simulink model "CurrentWithSim"  (R2022b)
settings: Solver=VariableStepAuto  StartTime=0.0  StopTime=20  RelTol=1e-3
PreLoadFcn:
  | openManipulatorParameters;
PostLoadFcn:
  | % Insert Communication Stuff Here
StartFcn:
  | myDxl.doEnableTorque(11);
  | myDxl.doEnableTorque(12);
  | myDxl.doEnableTorque(13);
  | myDxl.doEnableTorque(14);
  | myDxl.doEnableTorque(15);
StopFcn:
  | myDxl.doDisableTorque(11);
  | myDxl.doDisableTorque(12);
  | myDxl.doDisableTorque(13);
  | myDxl.doDisableTorque(14);
  | myDxl.doDisableTorque(15);
undefined symbols (not defined in the file): TsCtrl
libraries: slDxl_lib x12, OpenManipulatorLib x3, sm_lib x2, nesl_utility x1
CloseFcn:
  | myDxl.delete()
settings Model: Creator=scastro  LastModifiedBy=Boog
settings SolverCC: AlgebraicLoopSolver=TrustRegion  DecoupledContinuousIntegration=on  MinimalZcImpactIntegration=on
settings DataIOCC: ReturnWorkspaceOutputs=off
settings DebuggingCC: UnconnectedInputMsg=warning  UnconnectedOutputMsg=warning  UnconnectedLineMsg=warning  SFMachineParentedDataDiag=warning  ArithmeticOperatorsInVariantConditions=warning
settings ModelReferenceCC: EnableRefExpFcnMdlSchedulingChecks=on
settings SFSimCC: SimUseLocalCustomCode=off  CustomCodeUndefinedFunction=UseInterfaceOnly
settings RTWCC: RTWUseLocalCustomCode=off
settings ExplorerConfigSet: InternalSimMechanicsExplorerSettings="<ExplorerConfiguration><canonicalview>default</canonicalview><AnimationSetting><BasePlaybackSpeed>1.0</BasePlaybackSpeed><PlaybackSpeedFactor>1.0</PlaybackSpeedFactor></AnimationSetting><TilePanel><TileInfo><Tiles Columns=\"1\" Count=\"1\" Rows=\"1\"><Column Weight=\"1\"/><Row Weight=\"1\"/><Tile Height=\"1\" Width=\"1\" X=\"0\" Y=\"0\"/></Tiles></TileInfo><SceneInfo><SceneViewer><BGColor><R>0.60000002384185791</R><G>0.60000002384185791</G><B>0.60000002384185791</B></BGColor><Camera><DoPerspective>off</DoPerspective><Position><X>0.428752942017998073</X><Y>-0.712150369953937545</Y><Z>0.628314823463847372</Z></Position><Center><X>0.0455703138120887447</X><Y>0.0802507835591396851</Y><Z>0.153687090021758288</Z></Center><Up><X>-0.128866037345358619</X><Y>0.462960972240881619</Y><Z>0.876961049648547597</Z></Up><ViewLimDist>1</ViewLimDist><YLim>0.579070269035580121</YLim><XLim>0.64437894599448009</XLim></Camera></SceneViewer></SceneInfo></TilePanel><MechEditorPanel><Cameras/><GfxPanelCameraMap/><VideoCreator><PlaybackSpeedRatio>1.0</PlaybackSpeedRatio><FrameRate>30</FrameRate><VideoFormat>Motion JPEG AVI</VideoFormat><FrameSize>auto</FrameSize></VideoCreator></MechEditorPanel></ExplorerConfiguration>"

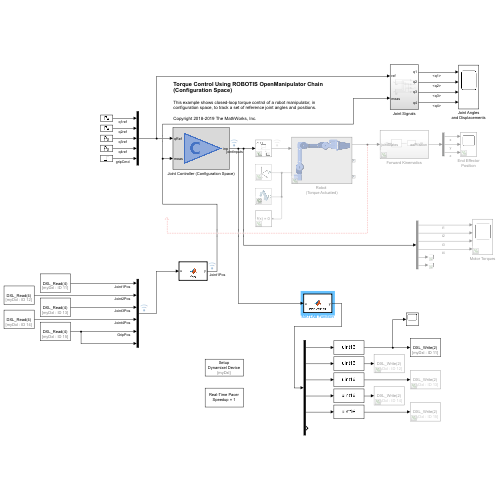
[thumbnail: Simulink's stored preview of the top-level diagram]
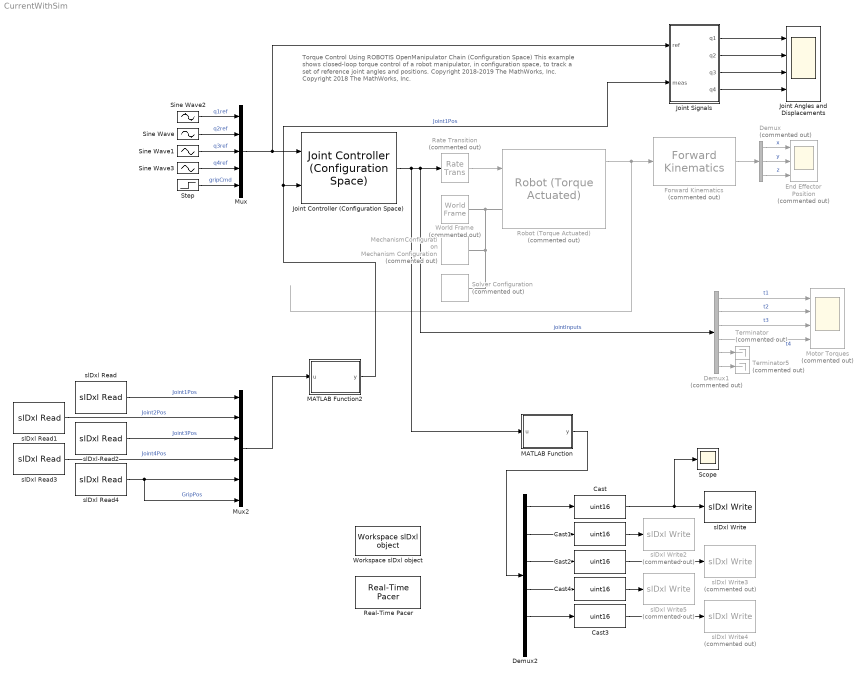
== system CurrentWithSim ==
  note: Torque Control Using ROBOTIS OpenManipulator Chain (Configuration Space)
      |
      | This example shows closed-loop torque control of a robot manipulator, in configuration space, to track a set of reference joint angles and positions.
      |
      | Copyright 2018-2019 The MathWorks, Inc.
      |
      | Copyright 2018 The MathWorks, Inc.
  Cast{,1..4} (5 alike) : DataTypeConversion  OutDataTypeStr=uint16  SaturateOnIntegerOverflow=off  RndMeth=Floor
  Demux : Demux  Commented=on  Outputs=3
  Demux1 : Demux  Commented=on  Outputs=6
  Demux2 : Demux  Outputs=6
  End Effector Position : Scope  Commented=on  NumInputPorts=3
  Forward Kinematics : OpenManipulatorLib/Forward Kinematics  Commented=on  SystemSampleTime=-1  VariantActivationTime=update diagram  Latency=0  AutoFrameSizeCalculation=off
  Joint Angles and Displacements : Scope  NumInputPorts=4
  Joint Controller (Configuration Space) : OpenManipulatorLib/Joint Controller (Configuration Space)  SystemSampleTime=-1  VariantControl=ctrlType==1  VariantActivationTime=update diagram  Latency=0  AutoFrameSizeCalculation=off
  Joint Signals : Subsystem
  MATLAB Function : MATLAB Function  TreatAsAtomicUnit=on
  MATLAB Function2 : MATLAB Function  TreatAsAtomicUnit=on
  MechanismConfiguration : sm_lib/Utilities/Mechanism Configuration  Commented=on  UniformGravity=Constant  GravityVector=[0 0 -9.80665]  GravityUnits=m/s^2  LinearizationDelta=0.001  JointModeTransitionNonlinearIterations=2
  Motor Torques : Scope  Commented=on  NumInputPorts=4
  Mux : Mux  Inputs=5
  Mux2 : Mux  Inputs=6
  Rate Transition : RateTransition  Commented=on
  Real-Time Pacer : slDxl_lib/Real-Time Pacer  simTimePerRealTime=1
  Robot (Torque Actuated) : OpenManipulatorLib/Robot  (Torque Actuated)  Commented=on  SystemSampleTime=-1  VariantActivationTime=update diagram  Latency=0  AutoFrameSizeCalculation=off
  Scope : Scope
  Sine Wave : Sin  Amplitude=pi/4  Frequency=0.6  SampleTime=TsCtrl
  Sine Wave1 : Sin  Amplitude=pi/4  Frequency=1.5  SampleTime=TsCtrl
  Sine Wave2 : Sin  Amplitude=2*pi/3  Frequency=0.4  SampleTime=TsCtrl
  Sine Wave3 : Sin  Amplitude=pi/3  SampleTime=TsCtrl
  Solver Configuration : nesl_utility/Solver Configuration  Commented=on  PhysicalDomain=network_engine_domain  SubClassName=solver  LeftPortType=input  RightPortType=generic  Tones=[]  Harmonics=[]  SimulateNoise=off  Profile=off  UseLocalSampling=off  EnableSwitchedLinearOptims=on  FrequencyDomain=off  UseCCode=off  RelTol=0.001  AbsTol=1e-06  MinStep=1e-09  ToWorkspace=off  RevertToSquareIcSolve=off  NumHomotopyIterations=100  PhasorMode=off  PhasorModeNumHarmonics=1  ConsistencySolver=NEWTON_FTOL  IndexReductionMethod=DerivativeReplacement  DoDC=off  ResidualTolerance=1e-09  ConsistencyTolSource=GLOBAL  ConsistencyAbsTol=0.001  ConsistencyRelTol=0.001  ConsistencyTolFactor=0.001  UseLocalSolver=off  LocalSolverChoice=NE_BACKWARD_EULER_ADVANCER  ResolveIndetEquations=on  FunctionEvalNumThread=1  LocalSolverSampleTime=0.001  DoFixedCost=off  MaxNonlinIter=3  MaxModeIter=2  ComputeImpulses=off  ImpulseIterations=2  LinearAlgebra=Sparse  LinearAlgebraNumThread=0  EquationFormulation=NE_TIME_EF  DelaysMemoryBudget=1024  AutomaticFiltering=on  FilteringTimeConstant=0.001  PartitionStorageMethod=AS_NEEDED  PartitionMemoryBudget=1024  PartitionMethod=FAST
  Step : Step  Time=5  SampleTime=TsCtrl
  Terminator : Terminator  Commented=on
  Terminator5 : Terminator  Commented=on
  Workspace slDxl object : slDxl_lib/Workspace slDxl object  slDxlVarName=Existing Object Handle #1  workspaceVarName=myDxl
  World Frame : sm_lib/Frames and Transforms/World Frame  Commented=on
  slDxl Read : slDxl_lib/slDxl Read  slDxlObject=Existing Object Handle #1  DXL_ID=11  DXL_ADDR=132  DXL_READ_SIZE=4  sampleT=Ts
  slDxl Read1 : slDxl_lib/slDxl Read  slDxlObject=Existing Object Handle #1  DXL_ID=12  DXL_ADDR=132  DXL_READ_SIZE=4  sampleT=Ts
  slDxl Read2 : slDxl_lib/slDxl Read  slDxlObject=Existing Object Handle #1  DXL_ID=13  DXL_ADDR=132  DXL_READ_SIZE=4  sampleT=Ts
  slDxl Read3 : slDxl_lib/slDxl Read  slDxlObject=Existing Object Handle #1  DXL_ID=14  DXL_ADDR=132  DXL_READ_SIZE=4  sampleT=Ts
  slDxl Read4 : slDxl_lib/slDxl Read  slDxlObject=Existing Object Handle #1  DXL_ID=15  DXL_ADDR=132  DXL_READ_SIZE=4  sampleT=Ts
  slDxl Write : slDxl_lib/slDxl Write  slDxlObject=Existing Object Handle #1  DXL_ID=11  DXL_ADDR=102  DXL_WRITE_SIZE=2  sampleT=Ts
  slDxl Write2 : slDxl_lib/slDxl Write  Commented=on  slDxlObject=Existing Object Handle #1  DXL_ID=12  DXL_ADDR=102  DXL_WRITE_SIZE=2  sampleT=Ts
  slDxl Write3 : slDxl_lib/slDxl Write  Commented=on  slDxlObject=Existing Object Handle #1  DXL_ID=13  DXL_ADDR=102  DXL_WRITE_SIZE=2  sampleT=Ts
  slDxl Write4 : slDxl_lib/slDxl Write  Commented=on  slDxlObject=Existing Object Handle #1  DXL_ID=15  DXL_ADDR=102  DXL_WRITE_SIZE=2  sampleT=Ts
  slDxl Write5 : slDxl_lib/slDxl Write  Commented=on  slDxlObject=Existing Object Handle #1  DXL_ID=14  DXL_ADDR=102  DXL_WRITE_SIZE=2  sampleT=Ts
  wires:
  Robot (Torque Actuated)/1 -> Forward Kinematics/1
  Sine Wave/1 -> Mux/2  "q2ref"
  Sine Wave1/1 -> Mux/3  "q3ref"
  Sine Wave2/1 -> Mux/1  "q1ref"
  Rate Transition/1 -> Robot (Torque Actuated)/1
  Mux/1 -> Joint Controller (Configuration Space)/1, Joint Signals/1(ref)
  Joint Signals/1(q1) -> Joint Angles and Displacements/1
  Joint Signals/2(q2) -> Joint Angles and Displacements/2
  Joint Signals/3(q3) -> Joint Angles and Displacements/3
  Joint Signals/4(q4) -> Joint Angles and Displacements/4
  Sine Wave3/1 -> Mux/4  "q4ref"
  Step/1 -> Mux/5  "gripCmd"
  Joint Controller (Configuration Space)/1 -> MATLAB Function/1(u), Demux1/1, Rate Transition/1  "jointInputs"
  Forward Kinematics/1 -> Demux/1
  Demux/1 -> End Effector Position/1  "x"
  Demux/2 -> End Effector Position/2  "y"
  Demux/3 -> End Effector Position/3  "z"
  Demux1/5 -> Terminator/1
  Demux1/4 -> Motor Torques/4  "t4"
  Demux1/3 -> Motor Torques/3  "t3"
  Demux1/2 -> Motor Torques/2  "t2"
  Demux1/1 -> Motor Torques/1  "t1"
  Demux1/6 -> Terminator5/1
  Demux2/1 -> Cast/1
  Cast/1 -> Scope/1, slDxl Write/1
  MATLAB Function/1(y) -> Demux2/1
  Cast1/1 -> slDxl Write2/1
  Cast2/1 -> slDxl Write3/1
  Cast3/1 -> slDxl Write4/1
  Cast4/1 -> slDxl Write5/1
  Demux2/5 -> Cast3/1
  Demux2/2 -> Cast1/1
  Demux2/3 -> Cast2/1
  Demux2/4 -> Cast4/1
  slDxl Read4/1 -> Mux2/6, Mux2/5  "GripPos"
  Mux2/1 -> MATLAB Function2/1(u)
  slDxl Read3/1 -> Mux2/4  "Joint4Pos"
  slDxl Read1/1 -> Mux2/2  "Joint2Pos"
  slDxl Read/1 -> Mux2/1  "Joint1Pos"
  slDxl Read2/1 -> Mux2/3  "Joint3Pos"
  MATLAB Function2/1(y) -> Joint Signals/2(meas), Joint Controller (Configuration Space)/2  "Joint1Pos"
  connections:
  Robot (Torque Actuated)/LConn1 -- Solver Configuration/RConn1 -- MechanismConfiguration/RConn1 -- World Frame/RConn1

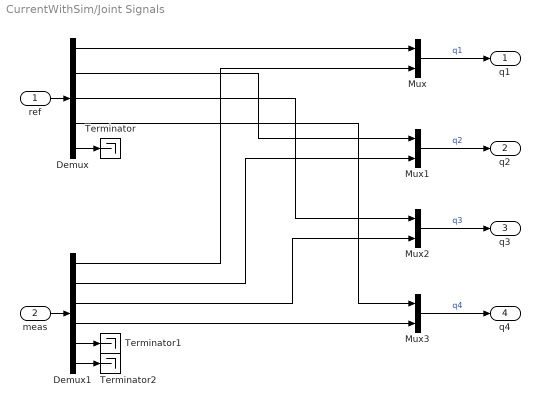
== system CurrentWithSim/Joint Signals ==
  ref : Inport
  meas : Inport  Port=2
  Demux : Demux  Outputs=5
  Demux1 : Demux  Outputs=6
  Mux{,1..3} (4 alike) : Mux  Inputs=2
  Terminator : Terminator
  Terminator1 : Terminator
  Terminator2 : Terminator
  q1 : Outport  VectorParamsAs1DForOutWhenUnconnected=off
  q2 : Outport  Port=2  VectorParamsAs1DForOutWhenUnconnected=off
  q3 : Outport  Port=3  VectorParamsAs1DForOutWhenUnconnected=off
  q4 : Outport  Port=4  VectorParamsAs1DForOutWhenUnconnected=off
  wires:
  Mux2/1 -> q3/1  "q3"
  ref/1 -> Demux/1
  Mux3/1 -> q4/1  "q4"
  Mux/1 -> q1/1  "q1"
  meas/1 -> Demux1/1
  Demux/1 -> Mux/1
  Demux1/1 -> Mux/2
  Mux1/1 -> q2/1  "q2"
  Demux/2 -> Mux1/1
  Demux1/2 -> Mux1/2
  Demux/3 -> Mux2/1
  Demux1/3 -> Mux2/2
  Demux1/4 -> Mux3/2
  Demux/4 -> Mux3/1
  Demux/5 -> Terminator/1
  Demux1/5 -> Terminator1/1
  Demux1/6 -> Terminator2/1

== matlab function CurrentWithSim/MATLAB Function2 ==
  data: u input; y output
function y = fcn(u)
y = (0.001534355386369.*u) - 3.14;

== matlab function CurrentWithSim/MATLAB Function ==
  data: u input; y output
function y = converter(u)
    current_A = 0.5714 .* u;
    y = current_A .* 1000 ./ 2.69;
